simulink library "Lib_Turbo_Nozzle_TMATS"  (R2012b)
settings: Solver=ode45  StartTime=0.0  StopTime=10.0  RelTol=1e-3
Description:
  | Thomas Modules
settings Model: Creator=jwchapm2  LastModifiedBy=jwchapm2

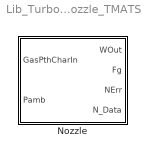
== system Lib_Turbo_Nozzle_TMATS ==
  Nozzle : Subsystem  mask(T-MATS: Nozzle Library Block){N_TArea_M=110.7, N_FL_M=0.00, X_N_TtVec2_M=[300 10000], T_N_TGArray_M=[1 1], X_N_PEQPaVec_M=[0 10000], T_N_CdThArray_M=[1 1], X_N_FARVec_M=[0; 0.0050; 0.0100; 0.0150; 0.0200; 0.0250; 0.0300], T_N_RtArray_M=[0.0686;    0.0686;    0.0686;    0.0686;    0.0686;    0.0686;    0.0686], Y_N_TtVec_M=[300 10000], T_N_MAP_gammaArray_M=[ 1.4 1.4 1.4 1.4 1.4 1.4 1.4; 1.4 1.4 1.4 1.4 1.4 1.4 1.4], T_N_CvArray_M=[0.990 0.990], iDesign_M=off, WDes_M=100}
      mask prompts: N_TArea_M "N_TArea_M - Nozzle Throat Area [in^2]"; N_FL_M "N_FL_M - Flow Loss Across Nozzle [%]"; X_N_TtVec2_M "X_N_TtVec2_M - Nozzle Total Temperature Vector (X-axis for TG calc)(ax1)"; T_N_TGArray_M "T_N_TGArray_M - Nozzle Thermal Growth Array (TG = f(Tt))(ax1)"; X_N_PEQPaVec_M "X_N_PEQPaVec_M - Nozzle PE/Pa Vector (X-axis) (bx1)"; T_N_CdThArray_M "T_N_CdThArray_M - Nozzle CdTh Array, Blockage Factor [frac] (CdTh = f(PEQPa)) (bx1)"; X_N_FARVec_M "X_N_FARVec_M - Nozzle Fuel to Air Ratio Vector (X-axis) (cx1)"; T_N_RtArray_M "T_N_RtArray_M - Nozzle Gas Constant, R, Array (R = f(FAR))(cx1)"; Y_N_TtVec_M "Y_N_TtVec_M - Nozzle Total Temperature Vector (Y-axis for Gamma calc)(dx1)"; T_N_MAP_gammaArray_M "T_N_MAP_gammaArray_M - Nozzle Map Gamma Array (Gamma = f(Tt,FAR))(dxc)"; T_N_CvArray_M "T_N_CvArray_M - Nozzle Cv Array (Cv = f(PEQPa)), PEQPa is defined under the General Tab(bx1)"; iDesign_M "iDesign_M - Drive nozzle flow to the design flow through NErr"; WDes_M "WDes_M - Design Flow [pps]"
      mask help: This block simulates the performance of a nozzle using basic thermodynamic equations, properties, and table lookups.
      mask Help: web(which('Turbo_TMATS_Noz.html'),'-helpbrowser')
      mask Callback iDesign_M: MSK_SEC_Enables_TMATS('iDesign_M',13,'en')

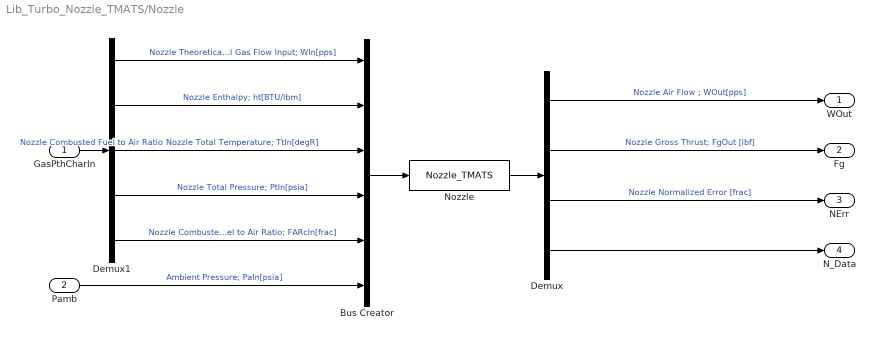
== system Lib_Turbo_Nozzle_TMATS/Nozzle ==
  GasPthCharIn : Inport
  Pamb : Inport  Port=2
  Bus Creator : BusCreator  Inputs=6
  Demux : Demux
  Demux1 : Demux  Outputs=5
  Nozzle : S-Function  FunctionName=Nozzle_TMATS  Parameters=N_TArea_M, N_FL_M, X_N_FARVec_M, T_N_RtArray_M, Y_N_TtVec_M, T_N_MAP_gammaArray_M, X_N_PEQPaVec_M, T_N_CdThArray_M, T_N_CvArray_M, T_N_TGArray_M, X_N_TtVec2_M, iDesign_M, WDes_M, gcs  EnableBusSupport=off
  WOut : Outport
  Fg : Outport  Port=2
  NErr : Outport  Port=3
  N_Data : Outport  Port=4
  wires:
  Demux1/4 -> Bus Creator/4  "Nozzle Total Pressure; PtIn[psia]"
  Pamb/1 -> Bus Creator/6  "Ambient Pressure; PaIn[psia]"
  Bus Creator/1 -> Nozzle/1
  Demux/2 -> Fg/1  "Nozzle Gross Thrust; FgOut [lbf]"
  Demux/1 -> WOut/1  "Nozzle Air Flow ; WOut[pps]"
  Nozzle/1 -> Demux/1
  Demux1/3 -> Bus Creator/3  "Nozzle Total Temperature; TtIn[degR]"
  Demux1/5 -> Bus Creator/5  "Nozzle Combusted Fuel to Air Ratio; FARcIn[frac]"
  Demux/4 -> N_Data/1
  GasPthCharIn/1 -> Demux1/1  "Nozzle Combusted Fuel to Air Ratio"
  Demux1/1 -> Bus Creator/1  "Nozzle Theoretical Gas Flow Input; WIn[pps]"
  Demux/3 -> NErr/1  "Nozzle Normalized Error [frac]"
  Demux1/2 -> Bus Creator/2  "Nozzle Enthalpy; ht[BTU/lbm]"
